simulink model "Sim_On_Off"  (R2020a)
settings: Solver=FixedStepAuto  StartTime=0.0  StopTime=800  FixedStep=0.1  RelTol=1e-3
settings Model: Creator=MK  LastModifiedBy=olive

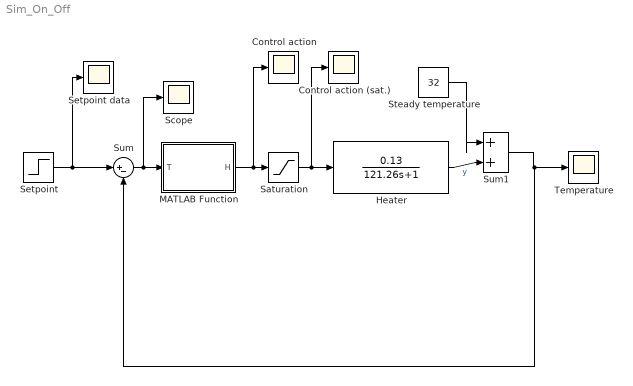
== system Sim_On_Off ==
  Control action : Scope
  Control action (sat.) : Scope
  Heater : TransferFcn  Numerator=0.13  Denominator=[121.26 1]
  MATLAB Function : MATLAB Function  TreatAsAtomicUnit=on
  "Saturation " : Saturate  UpperLimit=50  LowerLimit=-50
  Scope : Scope
  Setpoint : Step  Time=10  Before=32  After=36  SampleTime=0
  Setpoint data : Scope
  Steady temperature : Constant  Value=32
  Sum : Sum  Inputs=|+-
  Sum1 : Sum  Inputs=|++
  Temperature : Scope
  wires:
  Setpoint/1 -> Setpoint data/1, Sum/1
  Steady temperature/1 -> Sum1/1
  Heater/1 -> Sum1/2  "y"
  Sum1/1 -> Sum/2, Temperature/1
  "Saturation "/1 -> Control action (sat.)/1, Heater/1
  MATLAB Function/1(H) -> Control action/1, "Saturation "/1
  Sum/1 -> Scope/1, MATLAB Function/1(T)

== matlab function Sim_On_Off/MATLAB Function ==
  data: T input; H output
function H = control(T)

if T<0
    H = -50;
elseif T>0
    H = 50;
else
    H = 0;
end
